simulink model "Integration2022b_May06"  (R2022b)
settings: Solver=FixedStepAuto  StartTime=0.0  StopTime=inf  RelTol=1e-3
model workspace (MAT data in the model file):
  L = 4.165
  SL_ROS_VariableLengthArrays_MaxSizes : object (value not decoded)
  finalint = 0
  firstWarning = 1
  originalScenarioChecksum = '114339432DE22364D47BB28FC96DC10C'
values from neighbouring files (symbols this model uses):
  D = cross(B-A,C-A)    [HelperCalculateEgoRefPathInfo.m]
  data =     [Part_of_MCity.mat]    (also in curvedroad_Bhanu.mat; plotWPScript.m = [data, [out.x.Data(:, :, i); out.y.Data(:, :, i)]])
  x = [Vertices(Na,1) Vertices(:,1) Vertices(Nb,1)]    [HelperCalculateEgoRefPathInfo.m]    (also in HelperConvertDSPoseToSim3D.m = actor(1).Position(1); xpts.mat = [-29.9023190589 -34.2715935353 -19.4160603154 -19.4160603154)
  y = [Vertices(Na,2) Vertices(:,2) Vertices(Nb,2)]    [HelperCalculateEgoRefPathInfo.m]    (also in HelperConvertDSPoseToSim3D.m = actor(1).Position(2); VehicleOutputFcn.m = [x(1);x(2); x(3); x(4); x(5);x(6)]; ypts.mat = [-62.3254015256 -62.9079714558 -51.8391427821 -48.6350081661)
  z = zeros(1, length(interpX))    [HelperCalculateEgoRefPathInfo.m]
undefined symbols (not defined in the file or in its folder): MinVelocity, WB
libraries: ros2lib x13, mpcsigdimcheck_private x10, robotalgslib x1, mpclib x1, drivingvehiclecontroller x1, slpidlib x1
(part 3 of 5)

== matlab function Integration2022b_May06/BuckeyeLot Waypoints ==
  data: origin output; waypoints output
function [origin, waypoints] = fcn()

waypoints = [40.01521305598	-83.03187202052	229
40.01521322163	-83.03187211136	229
40.01521369926	-83.03187237033	229
40.0152143053	-83.03187268176	229
40.01521559418	-83.03187333109	229
40.01521705522	-83.0318740687	229
40.01521890093	-83.03187499475	229
40.01522126677	-83.03187620922	229
40.01522376357	-83.03187752424	229
40.01522693436	-83.03187916252	229
40.01523037713	-83.03188091942	229
40.01523440651	-83.03188299186	229
40.01523889274	-83.03188526667	229
40.01524237904	-83.03188703766	229
40.0152489772	-83.03189042263	229
40.01525450699	-83.0318932412	229
40.01526073314	-83.03189635526	229
40.01526699657	-83.03189951811	229
40.01527186155	-83.03190201932	229
40.015280801	-83.03190657434	229
40.01528807634	-83.03191025624	229
40.01529573611	-83.03191416025	229
40.0153037398	-83.03191818987	229
40.01531191961	-83.03192231971	229
40.0153212374	-83.03192705659	229
40.01533001373	-83.03193142778	229
40.01533949683	-83.03193620602	229
40.01534733224	-83.0319401166	229
40.01535607577	-83.0319445896	229
40.01536786231	-83.03195049094	229
40.01537798899	-83.03195561545	229
40.01538780584	-83.03196055965	229
40.01539517681	-83.03196424234	229
40.01540614703	-83.03196979803	229
40.0154183549	-83.03197587027	229
40.01542915249	-83.03198131587	229
40.01543939605	-83.03198643645	229
40.01544708561	-83.03199030719	229
40.01546057959	-83.03199712006	229
40.01547163575	-83.03200268625	229
40.0154821448	-83.03200793611	229
40.0154932675	-83.03201357949	229
40.01550182622	-83.03201784846	229
40.01551477273	-83.03202438112	229
40.01552559475	-83.03202977594	229
40.01553759261	-83.03203578543	229
40.01554863628	-83.03204128833	229
40.01555801577	-83.03204610684	229
40.01557129372	-83.03205278005	229
40.01558289136	-83.03205882874	229
40.0155939726	-83.03206436771	229
40.01560545366	-83.03207025111	229
40.01561472619	-83.03207500682	229
40.01562727451	-83.03208133221	229
40.01563805518	-83.03208676431	229
40.01564875652	-83.03209215271	229
40.01566054875	-83.03209804426	229
40.01567068279	-83.03210308312	229
40.01568226007	-83.03210884265	229
40.01569268087	-83.03211403066	229
40.01570307653	-83.0321191793	229
40.01571394869	-83.03212460218	229
40.01572211868	-83.03212859098	229
40.01573471957	-83.03213480769	229
40.01574473999	-83.03213975325	229
40.01575521671	-83.03214485209	229
40.01576458528	-83.03214961038	229
40.01577281371	-83.03215375888	229
40.01578532407	-83.03215992506	229
40.01579461904	-83.03216470123	229
40.01580431551	-83.03216949062	229
40.015811678	-83.03217299121	229
40.01582288391	-83.03217864033	229
40.01583168859	-83.03218291667	229
40.01584088607	-83.0321872971	229
40.01584939575	-83.03219146157	229
40.01585607553	-83.03219449739	229
40.01586551098	-83.03219835213	229
40.01587488028	-83.03220182921	229
40.01588340989	-83.032204311	229
40.01589141283	-83.03220583824	229
40.01589810845	-83.03220658227	229
40.01590727249	-83.03220656924	229
40.015914703	-83.03220563695	229
40.0159223544	-83.03220387611	229
40.01592969855	-83.03220114108	229
40.01593505652	-83.03219838995	229
40.01594206749	-83.03219385213	229
40.01594922416	-83.03218808843	229
40.0159546607	-83.03218246132	229
40.01595989328	-83.03217599392	229
40.01596354956	-83.0321707442	229
40.01596845733	-83.03216232631	229
40.01597227424	-83.03215461861	229
40.01597553537	-83.03214706029	229
40.01597855822	-83.03213892363	229
40.01598094675	-83.03213183334	229
40.01598389142	-83.03212275214	229
40.01598650142	-83.03211451517	229
40.01598856377	-83.03210787612	229
40.01599135684	-83.03209900865	229
40.01599233597	-83.03209597215	229
40.01599623811	-83.03208369583	229
40.01599859218	-83.03207628695	229
40.01600076324	-83.0320693128	229
40.016002502	-83.03206359906	229
40.0160041793	-83.03205823345	229
40.0160064141	-83.03205092722	229
40.01600818026	-83.03204507384	229
40.01600981096	-83.03203949986	229
40.01601114156	-83.03203530987	229
40.01601324352	-83.03202852053	229
40.01601536679	-83.03202123342	229
40.01601751415	-83.03201433116	229
40.01601968484	-83.0320072029	229
40.01602130953	-83.0320019914	229
40.01602404134	-83.03199287546	229
40.01602625551	-83.03198564744	229
40.01602835592	-83.03197877753	229
40.01603044795	-83.03197188272	229
40.01603212094	-83.03196639358	229
40.01603492202	-83.03195721071	229
40.01603712646	-83.03194991043	229
40.01603947305	-83.03194213828	229
40.01604177637	-83.03193466801	229
40.0160436105	-83.03192869357	229
40.01604647232	-83.0319193983	229
40.01604888376	-83.03191158231	229
40.01605117491	-83.03190429831	229
40.0160534885	-83.03189693822	229
40.01605506151	-83.03189189512	229
40.01605761386	-83.03188374716	229
40.01605944341	-83.03187791479	229
40.01606096522	-83.03187298586	229
40.01606234381	-83.03186860598	229
40.01606309443	-83.03186614964	229
40.01606426992	-83.03186244071	229
40.01606492827	-83.031860503	229
40.0160653701	-83.03185903609	229
40.01606562642	-83.03185827207	229
40.0160657086	-83.0318580822	229
40.0160656464	-83.03185826021	229
40.01606564447	-83.03185826119	229
40.01606565913	-83.03185826604	229
40.01606565849	-83.03185826432	229];

origin = waypoints(1,:);

end

== matlab function Integration2022b_May06/Controllers/Longitudinal Controllers/MJ Braking/Desired Accel Profile ==
  data: MaxBrakeFlag output; CurrVel input; DesiredDecel output; RelDist input; Dist1 output; StoppingDist input
function [MaxBrakeFlag,DesiredDecel,Dist1] = AccelProfile(CurrVel, RelDist, StoppingDist)
% time remaining = (current velocity) / (deceleration).
% desired velocity = (stopping distance - current distance) / time remaining.
Dist1 = RelDist;
Dist = Dist1 - StoppingDist;
if Dist1 <= 2
    MaxBrakeFlag = 1;
    DesiredDecel = 0;
else
    MaxBrakeFlag = 0;
    DesiredDecel = -min((CurrVel^2)/(2*Dist),3);
end
%     Dist = RelDist - (2.6850 + 3);
%     Decel = (CurrVel^2)/(2*Dist);
%     RemainingTime = CurrVel/Decel;
%     DesiredVel = Dist/RemainingTime; % DesiredVel = CurrVel/2

== stateflow chart Integration2022b_May06/Behavioural Planner/Behavioural Planner/Routing ==
  state InitialRoute
    en:
    NewRoute = 0;
  state Rerouting
    en:
    NewRoute = 1;
  (default) -> InitialRoute
  InitialRoute -> Rerouting : [ReRoute == 1]
  Rerouting -> InitialRoute : [ReRoute == 0]
  data: ReRoute input; NewRoute output

== matlab function Integration2022b_May06/Behavioural Planner/Behavioural Planner/StopSignPriority ==
  settings: updateMethod=DISCRETE
  data: ToAClearance output; SDist input; D2S input; ObjTracks input; egoSSPriority output; SceneTracks input; egoPose input; egoSpeed input; numSS output; SceneSpeed input; WB input; d output; flag input; flag output; midpoint input; midpoint output; egoExit output; egoEnter input; egoEnter output; process input; process output
function [ToAClearance, egoSSPriority, numSS, d, flag, midpoint, egoExit, egoEnter, process]  = StopSignPriority(SDist, D2S, ObjTracks, SceneTracks, egoPose, egoSpeed, SceneSpeed, WB, flag, midpoint, egoEnter, process)
% calculate covariance matrix outside, input to this block is modified with final, unique detections
egoPose = [-egoPose(2) egoPose(1) 90+egoPose(3)];
persistent SSPriority C1x C2y C3x C4y
% find stop signs + one of 2way or 4way or T-junction

% find number of signs (until we reach 0 valued columns)
numSS = 0;
for j = 1:length(SceneTracks(1,:))
    if any(SceneTracks(:,j))
        numSS = numSS + 1;
    end
end

% find number of cars
numObjects = 0;
for j = 1:length()
    if any(ObjTracks(:,j))
        numObjects = numObjects + 1;
    end
end


egoSSPriority = 1;
ToAClearance = 1;
ActorHeading = zeros(4,1);
actorExitang = zeros(4,1);
amax = 3;
ta = SceneSpeed/amax;
dd = 0.5*amax*(ta^2);
tcs = (19-dd)/SceneSpeed;
tt = ta + tcs;
tsafe = 1; % Adjusted for other conditions (e,g. weather, road condition ...)
ToAThreshold = tt + tsafe;
% tempPriority = zeros(numCars+1,1);
d = zeros(10, 5); % distance, velocity, time, location (wrt ego), exit (leaving ints)
Objang = zeros(10, 1);
% priorityTable = zeros(numCars+1, 5);
egoExitang = egoPose(3) - atan2d(midpoint(2)-egoPose(2),midpoint(1)-egoPose(1)); % 0 deg = straight , + = right
egoExitdist = sqrt((midpoint(2)-egoPose(2))^2+(midpoint(1)-egoPose(1))^2);

if abs(egoExitang) >= 135 && egoExitdist >= 10
    d(1,5) = 1; % ego left the ints
    egoEnter = 0;
    flag = 0;
elseif abs(egoExitang) >= 135 && egoExitdist <= 20 && egoExitdist >= 10
    d(1,5) = 1;
end

egoExit = d(1,5);


if (D2S <= SDist || egoEnter == 1) && process % && egoExitdist >= 12

    % [~, index] = min(abs(SceneTracks(1,:)'));
    if numSS > 0

        Vmd = [-egoSpeed*sind(egoPose(3)), egoSpeed*cosd(egoPose(3))];
        rot = [cosd(egoPose(3)) -sind(egoPose(3)); sind(egoPose(3)) cosd(egoPose(3))];
        

        % intersection region
        if flag == 0
            C1x = min(SceneTracks(1, 1:numSS)) - (WB + 3);
            C2y = min(SceneTracks(3, 1:numSS)) - (WB + 3);
            C3x = max(SceneTracks(1, 1:numSS)) + (WB + 3);
            C4y = max(SceneTracks(3, 1:numSS)) + (WB + 3);
            C1 = rot*[C1x; C2y] + egoPose(1:2)';
            C2 = rot*[C3x; C4y] + egoPose(1:2)';
            midpoint = (C1+C2)./2;
            
            % C1x = min(SceneTracks(1, 1:numSS)) - (WB + 3);
            % C2y = min(SceneTracks(3, 1:numSS)) - (WB + 3);
            % C3x = max(SceneTracks(1, 1:numSS)) + (WB + 3);
            % C4y = max(SceneTracks(3, 1:numSS)) + (WB + 3);
            % midpoint = [2*egoPose(1)-C4y-C2y; 2*egoPose(2)+C1x+C3x]./2;
        %   scatter(-SceneTracks(3,:)+egoPose(1),SceneTracks(1,:)+egoPose(2),'blue','filled')   
            % scatter(midpoint(1), midpoint(2), 'blue', 'filled')
            % rectangle('Position',[egoPose(1)-C4y egoPose(2)+C1x abs(C4y-C2y) abs(C3x-C1x)])
            flag = C1x;
        end

        midpoint_ego = rot'*(midpoint - egoPose(1:2)');
        
        % loop through num of cars (j)
    
        d(1,1) = sqrt((midpoint(1) - egoPose(1))^2 + (midpoint(2) - egoPose(2))^2);
        d(1,2) = egoSpeed;
        d(1,3) = d(1,1)/d(1,2);     %add ego TOA
        d(1,4) = 4; % 4 is the location of the ego vehicle itself
        
        % if d(1,1) <= 3
        %     ToAThreshold = 2;
        % else
        %     ToAThreshold = 6;
        % end

        if d(1,1) <= flag
            egoEnter = 1;
        end

    
        % loop through signs (vectorized)
        % if smallest dist 
        % d(:,3) -> TOA = v/dist
    
        if numObjects > 0
            for k = 1:numObjects
                d(k+1,1) = sqrt((midpoint_ego(2)-ObjTracks(3,k))^2+(midpoint_ego(1)-ObjTracks(1,k))^2); %sqrt((midpoint(1) - (-ObjTracks(3,k)+egoPose(1)))^2 + (midpoint(2) - (ObjTracks(1,k)+egoPose(2)))^2); 
                d(k+1,2) = sqrt((Vmd(1) - ObjTracks(2,k))^2 + (Vmd(2) - ObjTracks(4,k))^2);
                d(k+1,3) = d(k+1,1)/d(k+1,2); % TOA of other cars
                Objang(k) = atan2d(ObjTracks(1,k), -ObjTracks(3,k));
                                
                % Identify cars location (direction) wrt ego
                if Objang(k) <= 60
                    d(k+1,4) = 1; % 1 = E, 2 = N, 3 = W
                elseif Objang(k) > 60  && Objang(k) < 120
                    d(k+1,4) = 2; % 1 = E, 2 = N, 3 = W
                elseif Objang(k) >= 120
                    d(k+1,4) = 3; % 1 = E, 2 = N, 3 = W
                end

                % Identifying leaving cars
                
                % ActorHeading = atan2d(ObjTracks(2,k) - Vmd(1), -ObjTracks(4,k) - Vmd(2));
                ActorHeading(k) = atan2d(ObjTracks(2,k), ObjTracks(4,k));
                actorExitTheta = ActorHeading(k) - atan2d(midpoint_ego(1)-ObjTracks(1,k),midpoint_ego(2)-ObjTracks(3,k));
                if actorExitTheta > 180
                    actorExitang(k) = actorExitTheta - 360;
                elseif actorExitTheta < -180
                    actorExitang(k) = actorExitTheta + 360;
                else
                    actorExitang(k) = actorExitTheta;
                end
                %actorExitdist = sqrt((midpoint_ego(2)-ObjTracks(3,k))^2+(midpoint_ego(1)-ObjTracks(1,k))^2);
                

                if abs(actorExitang(k)) >= 135 && d(k+1,1) >= 10 
                    d(k+1,5) = 1; % left the ints
                else
                    d(k+1,5) = 0; % did not leave
                end

    
            end
    
            if numSS == 4 
                % Assign priorities based on rank TOA #1, before vehicle stops
                % d1 = d(d(:,1)~=0,:);
                [car, SSPriority] = sort(d(d(:,1)~=0 & d(:,5)==0));
                % priorityTable(:, 1:2) = [car, priority];
        
                tempPriority = find(SSPriority == 1); % ego SS priority
                if ~isempty(tempPriority)
                    egoSSPriority = tempPriority(1);
                end
            
            elseif numSS >= 1 && numSS < 4
                [car, SSPriority] = sort(d((d(:,4)==2 | d(:,4)==4) & d(:,5)==0));
                tempPriority = find(SSPriority == 1); % ego SS priority
                if ~isempty(tempPriority)
                    egoSSPriority = tempPriority(1);              
                end
                ToAClearance = double(all(d(d(:,1)~=0 & d(:,5)==0 & d(:,4)~=4,3) > ToAThreshold));
                
            end
    
        end
    end
    
    
    if ToAClearance == 1 && egoSSPriority == 1 && egoEnter == 1
        process = 0;
    else
        process = 1;
    end
    
    % if egoSpeed <= VelStop
    %     if SSPriority ~= 1
    %         % for all vehicles with higher priority
    %         % provide indicator signals to identify conflicts
    %         % check indicator signs/conflicts and update priority based on that
    %         % code to define leavingScene for other vehicles:
    %         % update priority table
    % 
    %     end
    % end
    
    
    
    

% elseif egoExit == 0
    

end

== matlab function Integration2022b_May06/Perception Pre-Processing/Subsystem/MATLAB Function ==
  data: CurrPosXY input; flag output; RefXY input; distance output
function [flag, distance] = fcn(CurrPosXY, RefXY)

    RefXYLast = [RefXY(end,1) RefXY(end,2)];
    
    distance = (RefXYLast(1) - CurrPosXY(1));
    if distance < 40
        flag = 1;
    else
        flag = 0;
    end
end

== matlab function Integration2022b_May06/Controllers/Longitudinal Controllers/New_Lisa ==
  data: distanceToScene input; referenceVelocity output; slowDownFlag input; safeStopDistance input; CurrVel input; desiredVelocity input; X_f input; X_f output; a_coeff input; a_coeff output
function [referenceVelocity, X_f, a_coeff] = VelocityProfiler(distanceToScene, slowDownFlag, safeStopDistance, CurrVel, desiredVelocity, X_f, a_coeff)

D2S = abs(distanceToScene);

% if ~brakingFlag
%     referenceVelocity = desiredVelocity;
% else
%     if DesiredDecel == 0
%         DesiredDecel = (CurrVel^2)/(2*dist);
%         referenceVelocity = sqrt(2*dist*DesiredDecel);
%     else
%         referenceVelocity = sqrt(2*max(dist - safeStopDistance, 0)*DesiredDecel);
%     end
% end
% 
% end

if ~slowDownFlag
    referenceVelocity = desiredVelocity;
    X_f = 0; 
elseif slowDownFlag && X_f == 0
    X_i = 0;
    X_f = D2S - 10; % Initial D2S at the moment when flag is raised (velocity poly starts from zero)
    
    P = [1, X_i, X_i^2, X_i^3, X_i^4, X_i^5;
         0, 1, 2*X_i, 3*X_i^2, 4*X_i^3, 5*X_i^4;
         0, 0, 2, 6*X_i, 12*X_i^2, 20*X_i^3;
         1, X_f, X_f^2, X_f^3, X_f^4, X_f^5;
         0, 1, 2*X_f, 3*X_f^2, 4*X_f^3, 5*X_f^4;
         0, 0, 2, 6*X_f, 12*X_f^2, 20*X_f^3];
    velocity = 5;       %mph
    % Initial Conditions
    Vx_i = CurrVel; 
    
    Ax_i = 0; 
    Vx_f = velocity / 2.237;
    Ax_f = -0.2; 
    Jx_i = 0;
    Jx_f = 0;
    InitialCond = [Vx_i; Ax_i; Jx_i; Vx_f; Ax_f; Jx_f];
    a_coeff = P\InitialCond;
    distCovered  = abs(X_f - (D2S - 10));
    referenceVelocity = max([1,distCovered,distCovered^2,distCovered^3,distCovered^4,distCovered^5]*a_coeff, 0);
else
    distCovered  = abs(X_f - (D2S - 10));
    referenceVelocity = max([1,distCovered,distCovered^2,distCovered^3,distCovered^4,distCovered^5]*a_coeff, 0);
    if (X_f - (D2S - 10)) <= 30
        velocity = 5;
        referenceVelocity = velocity / 2.237;
    end

end

== matlab function Integration2022b_May06/Subsystem/Velocity - Curvature ==
  data: desiredVelocity input; referenceVelocity output; curveMinThreshold input; curvature input
function referenceVelocity = velocityCurveCalculation(desiredVelocity,curveMinThreshold, curvature)

    if abs(curvature) >= 0 && abs(curvature) <= curveMinThreshold
        referenceVelocity = desiredVelocity;
    else
        r = 1/abs(curvature);
        referenceVelocity = min(desiredVelocity, sqrt(9.81*r*0.9*0.4));
    end

== matlab function Integration2022b_May06/Subsystem/Curvature Calculation ==
  data: RefXY input; curvatureAhead output; SlowdownDistance input; minimumCurvatureThreshold input; cumulativeDistance output
function [curvatureAhead, cumulativeDistance] = CurvatureCalculation(RefXY, SlowdownDistance, minimumCurvatureThreshold)

% minimumCurvatureThreshold: curvature value above which it is considered
% straight, not curved path

DX = gradient(RefXY(:, 1));
D2X = gradient(DX);
DY = gradient(RefXY(:,2));
D2Y = gradient(DY);
curvature = (DX.*D2Y - DY.*D2X) ./(DX.^2+DY.^2).^(3/2);

% Calculate Distance Vector
distanceMatrix = squareform(pdist(RefXY));
distanceSteps = zeros(length(RefXY)-1,1);
for i = 2:length(RefXY)
    distanceSteps(i-1,1) = distanceMatrix(i,i-1);
end
totalDistance = sum(distanceSteps); % Total distance travelled along reference path
cumulativeDistance = cumsum([0; distanceSteps]); % Distance for each waypoint

% Curvature Ahead Calculation
st = 0;
en = 1;
j1 = 1;
CurveInfo = zeros(length(curvature),7); % [startX startY endX endY MaxCurve startidx endidx]

for j = 1:length(curvature)
    if abs(curvature(j)) >= minimumCurvatureThreshold
        if abs(curvature(j)) >= CurveInfo(j1,5)
            CurveInfo(j1,5) = abs(curvature(j));
        end
        if st == 0
            CurveInfo(j1,1:2) = [RefXY(j,1) RefXY(j,2)]; % Startpoint
            CurveInfo(j1,6) = j;
            st = 1;
            en = 0;
        end
    elseif (abs(curvature(j)) < minimumCurvatureThreshold) && (en == 0)
            CurveInfo(j1,3:4) = [RefXY(j,1) RefXY(j,2)]; % Endpoint
            CurveInfo(j1,7) = j;
            j1 = j1+1;
            st = 0;
            en = 1;
    end
    if (j == length(curvature)) && (en == 0)
           CurveInfo(j1,3:4) = [RefXY(j,1) RefXY(j,2)]; % Endpoint
            CurveInfo(j1,7) = j;
            j1 = j1+1;
            st = 0;
            en = 1;
    end
end

j2 = 1;
curvatureAhead = zeros(length(curvature),1);
if j1 > 1
    for j = 1:length(cumulativeDistance)
        if (cumulativeDistance(j) >= (cumulativeDistance(CurveInfo(j2, 6)) - SlowdownDistance)) && (cumulativeDistance(j) < cumulativeDistance(CurveInfo(j2,7)))
            curvatureAhead(j) = CurveInfo(j2,5);
        elseif (cumulativeDistance(j) >= cumulativeDistance(CurveInfo(j2,7))) && (j2 < j1-1)
            curvatureAhead(j) = CurveInfo(j2,5);
            j2 = j2+1;
        else
            curvatureAhead(j) = curvature(j);
        end
    end
end

== matlab function Integration2022b_May06/Subsystem/Reference Pose Search ==
  data: RefXY input; currentPose input; referenceCurvature input; curvature output; cumulativeDistance input; currentDistanceTravelled output; referencePoses output; positionError output
function [curvature, currentDistanceTravelled, referencePoses, positionError] = referencePoseSearch(RefXY, currentPose, referenceCurvature, cumulativeDistance)

dist = zeros(length(RefXY),1);
for j = 1:length(RefXY)
    dist(j) = norm(currentPose(1:2) - RefXY(j,1:2));
end

[~, ind] = mink(dist,2);

if ind(1) > ind(2)
    ind = [ind(2); ind(1)];
end

curvature = referenceCurvature(ind(1));
currentDistanceTravelled = cumulativeDistance(ind(1));

referencePoses = zeros(1, 2);
m = 0; mm = 0; b = 0; bb = 0;
m = (RefXY(ind(1),2) - RefXY(ind(2),2))/(RefXY(ind(1),1) - RefXY(ind(2),1));
if m == 1e6
    referencePoses = [RefXY(ind(1),1) currentPose(2)];
elseif m == 1e-6
    referencePoses = [currentPose(1) RefXY(ind(1),2)];
else
    b = RefXY(ind(1),2) - m*RefXY(ind(1),1);
    mm = -1/m;
    bb = currentPose(2) - mm*currentPose(1);
    referencePoses(1:2) = [(b-bb)/(mm-m) m*((b-bb)/(mm-m)) + b];

end
positionError = norm(referencePoses(1:2) - currentPose(1:2));

== matlab function Integration2022b_May06/Controllers/Longitudinal Controllers/Longitduinal Controller/MATLAB Function2 ==
  data: distance2Scene input; Accel output; AccelCmd input; DecelCmd input; safeStop input; slowDownFlag input; Decel output; holdBrakeFlag input
function [Accel, Decel] = fcn(distance2Scene, AccelCmd, DecelCmd, safeStop, slowDownFlag, holdBrakeFlag)

if (distance2Scene <= safeStop && slowDownFlag == 1) || holdBrakeFlag == 1
    Accel = 0;
    Decel = -3;
else
    Accel = AccelCmd;
    Decel = DecelCmd;
end

== matlab function Integration2022b_May06/Controllers/Longitudinal Controllers/ACC Block/MATLAB Function ==
  data: ACC_Acceleration input; acceleration output; deceleration output
function [acceleration, deceleration] = fcn(ACC_Acceleration)
    
    if ACC_Acceleration > 0
        acceleration = ACC_Acceleration; 
        deceleration = 0;

    elseif ACC_Acceleration < 0
        acceleration = 0; 
        deceleration = ACC_Acceleration;

    else
        acceleration = 0;
        deceleration = 0;
    end
end

== matlab function Integration2022b_May06/Behavioural Planner/Traffic Sign Priority ==
  settings: updateMethod=DISCRETE
  data: Clear2Go output; SDist input; distance2Scene input; CurrentPose input; currentVelocity input; SceneSpeed input; transitionDistance input; matrixA input; sceneId input; signPose input
function Clear2Go = TrafficSignAssist(SDist, distance2Scene, CurrentPose, currentVelocity, SceneSpeed, transitionDistance, matrixA, sceneId, signPose)

% Intersection zones only
averageAcceleration = 3;
accelerationTime = SceneSpeed/averageAcceleration;
accelerationDistance = 0.5*averageAcceleration*(accelerationTime^2);
timeConstantSpeed = (transitionDistance - accelerationDistance)/SceneSpeed;
timeTotal = accelerationTime + timeConstantSpeed;
timeSafe = 1;
timeOfArrivalThreshold = timeTotal + timeSafe;
validValuesA = matrixA((matrixA(:,2) >= 1 & matrixA(:,2) <= 4) | matrixA(:,2) == 6,:);

d = zeros(8, 5);                                                            % distance, velocity, time, location, exit (leaving intersection)
% priorityTable = zeros(numCars+1, 5);
% egoExitAngle = CurrentPose(3) - atan2d(midpoint(2)-CurrentPose(2),midpoint(1)-CurrentPose(1)); % 0 deg = straight , + = right
% egoExitDistance = sqrt((midpoint(2)-CurrentPose(2))^2+(midpoint(1)-CurrentPose(1))^2);

if abs(egoExitAngle) >= 135 && egoExitDistance >= 10
    d(1,5) = 1; % ego left the ints
    egoEnter = 0;
    flag = 0;
elseif abs(egoExitAngle) >= 135 && egoExitDistance <= 20 && egoExitDistance >= 10
    d(1,5) = 1;
end

egoExit = d(1,5);

if ~isempty(validValuesA)
    objectAngle = validValuesA(:, 9);                                       % objectCourse from matrixA
    objectHeading = 90 - objectAngle;                                       % conversion to local coordinates
    if objectHeading < -180
       objectHeading = objectHeading + 360;
    elseif abs(objectHeading) == 180
       objectHeading = abs(objectHeading);
    end

% for intersection zones
if sceneId == (distance2Scene <= SDist || egoEnter == 1) && process % && egoExitdist >= 12

    % [~, index] = min(abs(SceneTracks(1,:)'));

    % if numSS > 0

    Vmd = [-currentVelocity*sind(CurrentPose(3)), currentVelocity*cosd(CurrentPose(3))];
    rot = [cosd(CurrentPose(3)) -sind(CurrentPose(3)); sind(CurrentPose(3)) cosd(CurrentPose(3))];
    

    % intersection region
    if flag == 0
        midpoint = [intersectionLength/sqrt(2) * cosd(currentPose(3) + 45), intersectionLength/sqrt(2) * sind(currentPose(3) + 45)];

        flag = distance2Scene - 10;
    end

    midpoint_ego = rot'*(midpoint - CurrentPose(1:2)');
    
    % loop through num of cars (j)

    d(1,1) = distance2Scene + ;
    d(1,2) = currentVelocity;
    d(1,3) = d(1,1)/d(1,2);                                                 % ego vehicle time o arrival at scene / intersection
    d(1,4) = 4;                                                             % 4 is the location of the ego vehicle itself
    
    % if d(1,1) <= 3
    %     ToAThreshold = 2;
    % else
    %     ToAThreshold = 6;
    % end

    if d(1,1) <= flag
        egoEnter = 1;
    end



    % loop through signs (vectorized)
    % if smallest dist 
    % d(:,3) -> TOA = v/dist
% determine: midpoint
    if numDynamicObjects > 0
        for k = 1:size(validValuesA(1))
            
            % theta = atan2d(validValuesA(k, 4), validValuesA(k, 3));
            % beta = theta + CurrentPose(3) - 90;
            objectAngle = validValuesA(:, 9);                                       % objectCourse from matrixA
            objectHeading = 90 - objectAngle;                                       % conversion to local coordinates
            if objectHeading < -180
               objectHeading = objectHeading + 360;
            elseif abs(objectHeading) == 180
               objectHeading = abs(objectHeading);
            end

            objectVector = norm([validValuesA(k, 4), validValuesA(k, 3)]);
            % xObject = objectVector*cosd(beta);
            % yObject = objectVector*sind(beta);
            dynamicObjectPose(k) = [xObject + CurrentPose(1), yObject + CurrentPose(2)];

            d(k+1,1) = sqrt((midpoint_ego(2)-ObjTracks(3,k))^2+(midpoint_ego(1)-ObjTracks(1,k))^2); %sqrt((midpoint(1) - (-ObjTracks(3,k)+egoPose(1)))^2 + (midpoint(2) - (ObjTracks(1,k)+egoPose(2)))^2); 
            d(k+1,2) = sqrt((Vmd(1) - ObjTracks(2,k))^2 + (Vmd(2) - ObjTracks(4,k))^2);
            d(k+1,3) = d(k+1,1)/d(k+1,2); % TOA of other cars
            objectAngle(k) = atan2d(ObjTracks(1,k), -ObjTracks(3,k));
                            
            % Identify cars location (direction) wrt ego
            if objectAngle(k) <= 60
                d(k+1,4) = 1; % 1 = E, 2 = N, 3 = W
            elseif objectAngle(k) > 60  && objectAngle(k) < 120
                d(k+1,4) = 2; % 1 = E, 2 = N, 3 = W
            elseif objectAngle(k) >= 120
                d(k+1,4) = 3; % 1 = E, 2 = N, 3 = W
            end

            % Identifying leaving objects (pedestrian/car)
            
            % ActorHeading = atan2d(ObjTracks(2,k) - Vmd(1), -ObjTracks(4,k) - Vmd(2));
            ActorHeading(k) = atan2d(ObjTracks(2,k), ObjTracks(4,k));
            actorExitTheta = ActorHeading(k) - atan2d(midpoint_ego(1)-ObjTracks(1,k),midpoint_ego(2) - ObjTracks(3,k));
            if actorExitTheta > 180
                actorExitang(k) = actorExitTheta - 360;
            elseif actorExitTheta < -180
                actorExitang(k) = actorExitTheta + 360;
            else
                actorExitang(k) = actorExitTheta;
            end
            %actorExitdist = sqrt((midpoint_ego(2)-ObjTracks(3,k))^2+(midpoint_ego(1)-ObjTracks(1,k))^2);
            

            if abs(actorExitang(k)) >= 135 && d(k+1,1) >= 10 
                d(k+1,5) = 1; % left the ints
            else
                d(k+1,5) = 0; % did not leave
            end


        end

        if numSS == 4 
            % Assign priorities based on rank TOA #1, before vehicle stops
            % d1 = d(d(:,1)~=0,:);
            [car, SSPriority] = sort(d(d(:,1)~=0 & d(:,5)==0));
            % priorityTable(:, 1:2) = [car, priority];
    
            tempPriority = find(SSPriority == 1); % ego SS priority
            if ~isempty(tempPriority)
                egoSSPriority = tempPriority(1);
            end
        
        elseif numSS >= 1 && numSS < 4
            [car, SSPriority] = sort(d((d(:,4)==2 | d(:,4)==4) & d(:,5)==0));
            tempPriority = find(SSPriority == 1); % ego SS priority
            if ~isempty(tempPriority)
                egoSSPriority = tempPriority(1);              
            end
            ToAClearance = double(all(d(d(:,1)~=0 & d(:,5)==0 & d(:,4)~=4,3) > timeOfArrivalThreshold));
               
        end
    end
    
    
    if ToAClearance == 1 && egoSSPriority == 1 && egoEnter == 1
        process = 0;
    else
        process = 1;
    end
    
    % if egoSpeed <= VelStop
    %     if SSPriority ~= 1
    %         % for all vehicles with higher priority
    %         % provide indicator signals to identify conflicts
    %         % check indicator signs/conflicts and update priority based on that
    %         % code to define leavingScene for other vehicles:
    %         % update priority table
    % 
    %     end
    % end
    
    

    

% elseif egoExit == 0
    

end

== matlab function Integration2022b_May06/Controllers/Longitudinal Controllers/Profile Generator/Profile Generator ==
  data: distanceToScene input; referenceVelocity output; slowDownFlag input; safeStopDistance input; CurrVel input; desiredVelocity input; X_f input; X_f output; a_coeff input; a_coeff output
function [referenceVelocity, X_f, a_coeff] = fcn(distanceToScene, slowDownFlag, safeStopDistance, CurrVel, desiredVelocity, X_f, a_coeff)

D2S = abs(distanceToScene);

% if ~brakingFlag
%     referenceVelocity = desiredVelocity;
% else
%     if DesiredDecel == 0
%         DesiredDecel = (CurrVel^2)/(2*dist);
%         referenceVelocity = sqrt(2*dist*DesiredDecel);
%     else
%         referenceVelocity = sqrt(2*max(dist - safeStopDistance, 0)*DesiredDecel);
%     end
% end
% 
% end

if ~slowDownFlag
    referenceVelocity = desiredVelocity;
    X_f = 0; 
elseif slowDownFlag && X_f == 0
    X_i = 0;
    X_f = D2S; % Initial D2S at the moment when flag is raised (velocity poly starts from zero)
    
    P = [1, X_i, X_i^2, X_i^3, X_i^4, X_i^5;
         0, 1, 2*X_i, 3*X_i^2, 4*X_i^3, 5*X_i^4;
         0, 0, 2, 6*X_i, 12*X_i^2, 20*X_i^3;
         1, X_f, X_f^2, X_f^3, X_f^4, X_f^5;
         0, 1, 2*X_f, 3*X_f^2, 4*X_f^3, 5*X_f^4;
         0, 0, 2, 6*X_f, 12*X_f^2, 20*X_f^3];
    
    % Initial Conditions
    Vx_i = CurrVel; 
    Ax_i = 0; 
    Vx_f = 0.3;
    Ax_f = -0.2; 
    Jx_i = 0;
    Jx_f = 0;
    InitialCond = [Vx_i; Ax_i; Jx_i; Vx_f; Ax_f; Jx_f];
    a_coeff = P\InitialCond;
    distCovered  = abs(X_f - D2S);
    referenceVelocity = max([1,distCovered,distCovered^2,distCovered^3,distCovered^4,distCovered^5]*a_coeff, 0);
else
    distCovered  = abs(X_f - D2S);
    referenceVelocity = max([1,distCovered,distCovered^2,distCovered^3,distCovered^4,distCovered^5]*a_coeff, 0);
    
end

end

== matlab function Integration2022b_May06/Calculate distance func3 ==
  data: startpoint input; curpos input; onoff output; entercriteria input; dif output
function [onoff, dif] = fcn(startpoint,curpos, entercriteria)

xdis = curpos(1,1)-startpoint(1,1);
ydis = curpos(1,2)-startpoint(1,2);
distance = sqrt(xdis^2+ydis^2);
dif=distance;
if (distance<entercriteria||abs(xdis)<1)
    onoff = 1;
else 
    onoff = 0;
end

== matlab function Integration2022b_May06/Create Parking Wp2 ==
  data: destinationpos input; angled_parking_wp output; ref_wp output; parking_angle input; arc_angle input; enter_dis input; start_steer_dis input; xref input; yref input; startpt output; curpos input; steerpto output; midsteerpt_o output; entrypt output; destpto output; data input
function [angled_parking_wp, ref_wp, startpt,steerpto,midsteerpt_o,entrypt, destpto] = fcn(destinationpos, parking_angle, arc_angle, enter_dis, start_steer_dis, xref, yref, curpos, data)


destpt = [destinationpos(1) , destinationpos(2)]    % parking point

% calculate stright line when entering the parking lot to stop

angle_deg = parking_angle; % assume lot is 30 degree
angle_rad = deg2rad(angle_deg); % radius
slope = tan(angle_rad); % stright line slope
distance = enter_dis; % entering distance
enterdestpt=calculatePointQ(destpt, slope, distance); % enter point

% find the arc
% find circle center first
% draw a opposite direction slope
arc_rad=deg2rad(arc_angle);
slope2= -tan(arc_rad)
radius=4.8         % car minimum turning radius
[arccenterx, arccentery]=findPointOnLineWithDistance(enterdestpt(1),enterdestpt(2), slope2, radius);

% arc degree
acr_degrees = arc_angle; % degree
% find the point 30degree from entering point as steering point
[steeringptx_mid, steeringpty_mid] = findPointAtAngle(arccenterx, arccentery, enterdestpt(1),enterdestpt(2), acr_degrees/2); % steering point
[steeringptx, steeringpty] = findPointAtAngle(arccenterx, arccentery, enterdestpt(1),enterdestpt(2), acr_degrees); % steering point

x_start=steeringptx;
y_start=steeringpty-start_steer_dis; %% stright line

start_pt=[x_start,y_start];
steerpt=[steeringptx,steeringpty];
mid_steerpt=[steeringptx_mid, steeringpty_mid];
entry_point=enterdestpt;
waypoints = [start_pt; steerpt;mid_steerpt;entry_point; destpt];
t = linspace(0, 1, length(waypoints));
ti = linspace(0, 1, 100);
spline_x = interp1(t, waypoints(:,1), ti, 'pchip');
spline_y = interp1(t, waypoints(:,2), ti, 'pchip');
waypoints_x = [spline_x(1,:)];
waypoints_y = [spline_y(1,:)];
waypoints= [waypoints_x;waypoints_y];
startpt=start_pt;
steerpto=steerpt;
midsteerpt_o=mid_steerpt;
entrypt=entry_point;
destpto=destpt;
% Calculate waypoints, separate into three portion
% Start to steering point

% all waypoints
angled_parking_wp = waypoints';
xref = xref;
yref = yref;

% new_xref = [xref(:); xref(end)];
% new_yref = [yref(:); yref(end)];
new_xref = [xref(:)];
new_yref = [yref(:)];
ref_wp = [new_xref(:), new_yref(:)];

function qpoint = calculatePointQ(p, slope, distance)
    x1 = p(1);
    y1 = p(2);

    delta_x = sqrt(distance^2 / (1 + slope^2));
    delta_y = slope * delta_x;
    if slope < 0
        delta_y = -delta_y; 
    end

    x2_2 = x1 - delta_x;
    y2_2 = y1 - delta_y;
    qpoint = [x2_2, y2_2];

end

function arcend = calculateCirclePoints(Q, angle_deg, radius)
    x_q = Q(1);
    y_q = Q(2);

    angle_rad = deg2rad(angle_deg);
    angle_rad_new = atan2(y_q, x_q) - angle_rad; % atan2 计算反正切角度

    x_new = radius * cos(angle_rad_new);
    y_new = radius * sin(angle_rad_new);
    arcend=[x_new, y_new];


end

function [x_c, y_c] = findCircleCenter(x1, y1, radius)
    syms x_c y_c;
    eqn1 = (x1 - x_c)^2 + (y1 - y_c)^2 == radius^2;
    eqn2 = x_c^2 + y_c^2 == 0; 

    sol = solve([eqn1, eqn2], [x_c, y_c]);

    x_c = double(sol.x_c);
    y_c = double(sol.y_c);
end


function [x2, y2] = findPointOnLineWithDistance(x1, y1, m, d)
    c = y1 - m * x1;

    x2 = x1 + d / sqrt(1 + m^2);
    y2 = y1 + m * d / sqrt(1 + m^2);
end

function [x_B, y_B] = findPointAtAngle(x_c, y_c, x_A, y_A, angle_degrees)
    r = sqrt((x_A - x_c)^2 + (y_A - y_c)^2);
    
    theta = atan2d(y_A - y_c, x_A - x_c);
    
    theta_prime = theta + angle_degrees;
    
    theta_prime_rad = deg2rad(theta_prime);
    
    x_B = x_c + r * cos(theta_prime_rad);
    y_B = y_c + r * sin(theta_prime_rad);
end

function [x_2, y_2] = findPointBelowLine(x_1, y_1, m, b, d)
    if isinf(m)
        x_2 = x_1;
        y_2 = y_1 - d;
    else
        x_2 = (y_1 - b + m * x_1 - d * sqrt(1 + m^2)) / m;
        y_2 = m * x_2 + b;
    end
end

function points = evenlyDistributePoints(x_a, y_a, x_b, y_b, n)
    delta_x = x_b - x_a;
    delta_y = y_b - y_a;
    
    step_x = delta_x / (n + 1);
    step_y = delta_y / (n + 1);
    
    points = zeros(n, 2);
    
    for i = 1:n
        points(i, 1) = x_a + i * step_x; 
        points(i, 2) = y_a + i * step_y; 
    end
    
end
function points = evenlyDistributePointsOnCircle(x_c, y_c, x_d, y_d, radius, n)
    theta_step = 2 * pi / n;
    
    points = zeros(n, 2);
    
    for i = 1:n
        theta = (i - 1) * theta_step;
        points(i, 1) = x_c + radius * cos(theta); 
        points(i, 2) = y_c + radius * sin(theta); 
    end
    
end

function points = evenlyDistributePointsOnArc(center, radius, start_point, end_point, n)
    x_o = center(1);
    y_o = center(2);
    x1 = start_point(1);
    y1 = start_point(2);
    x2 = end_point(1);
    y2 = end_point(2);
    
    start_theta = atan2(y1 - y_o, x1 - x_o);
    end_theta = atan2(y2 - y_o, x2 - x_o);
    
    points = evenlyDistributePointsOnArcHelper(x_o, y_o, radius, start_theta, end_theta, n);
    

end

function points = evenlyDistributePointsOnArcHelper(x_o, y_o, r, start_theta, end_theta, n)
    delta_theta = (end_theta - start_theta) / n;
    
    points = zeros(n, 2);
    
    for i = 1:n
        theta_i = start_theta + (i - 1) * delta_theta;
        x_i = x_o + r * cos(theta_i);
        y_i = y_o + r * sin(theta_i);
        points(i, :) = [x_i, y_i];
    end
end


end

== matlab function Integration2022b_May06/MATLAB Function2 ==
  data: wpref input; wpparking input; parkornot input; final_wp output
function final_wp = fcn(wpref, wpparking,parkornot)

if(parkornot)
    final_wp = wpparking;
else
    final_wp = wpref;
end
